simulink model "stand_IM"  (R2024a)
settings: Solver=ode45  StartTime=0.0  StopTime=10.0  RelTol=1e-3  EnableMultiTasking=on
values from neighbouring files (symbols this model uses):
  fn = 50    [stand_final.m]
  pp = 2    [stand_final.m]
  Un = 23.4    [stand_final.m]
libraries: General x35, Math x19, MotorControl x3, Control x3, Basic x2, StateControl x2, Filter x1
settings Model: Creator=hgrabner  LastModifiedBy=adminLab
settings SolverCC: AlgebraicLoopSolver=TrustRegion
settings DataIOCC: LimitDataPoints=on  SaveFormat=Array  SignalLoggingSaveFormat=ModelDataLogs  ReturnWorkspaceOutputs=off
settings OptimizationCC: ExpressionDepthLimit=2147483647  InitFltsAndDblsToZero=on  LifeSpan=inf
settings DebuggingCC: UnderspecifiedInitializationDetection=Classic  MergeDetectMultiDrivingBlocksExec=none  SolverPrmCheckMsg=warning  FcnCallInpInsideContextMsg=warning  UnconnectedInputMsg=warning  UnconnectedOutputMsg=warning  UnconnectedLineMsg=warning  StateNameClashWarn=warning  SFUnexpectedBacktrackingDiag=warning  SFNoUnconditionalDefaultTransitionDiag=warning  SFExecutionAtInitializationDiag=none  ArithmeticOperatorsInVariantConditions=warning
settings HardwareCC: ProdBitPerPointer=32  ProdBitPerSizeT=32  ProdBitPerPtrDiffT=32  ProdLargestAtomicFloat=None  ProdIntDivRoundTo=Undefined  ProdEndianess=Unspecified  ProdWordSize=32  ProdHWDeviceType=32-bit Generic
settings ModelReferenceCC: EnableRefExpFcnMdlSchedulingChecks=on  PropagateSignalLabelsOutOfModel=off
settings SFSimCC: SimUseLocalCustomCode=off  CustomCodeUndefinedFunction=UseInterfaceOnly
settings RTWCC: RTWUseLocalCustomCode=off  GPUComputeCapability=3.5  DLArmComputeVersion=19.05
settings CodeAppCC: StateflowObjectComments=on
settings GRTTargetCC: TargetLangStandard=C89/C90 (ANSI)  CombineOutputUpdateFcns=off  GRTInterface=on
settings ConfigComp: CovMetricSettings=dw  CovSaveCumulativeToWorkspaceVar=on  CovSaveSingleToWorkspaceVar=on  CovExternalEMLEnable=off

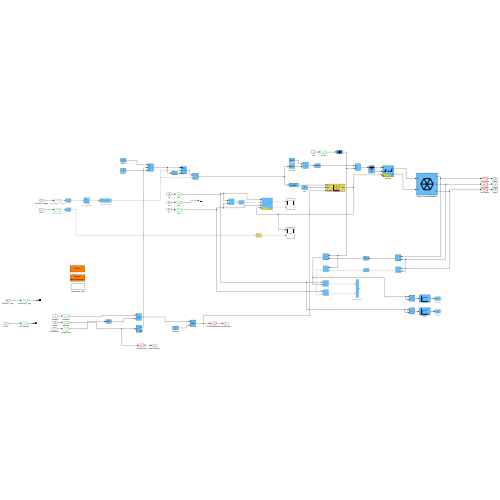
[thumbnail: Simulink's stored preview of the top-level diagram]
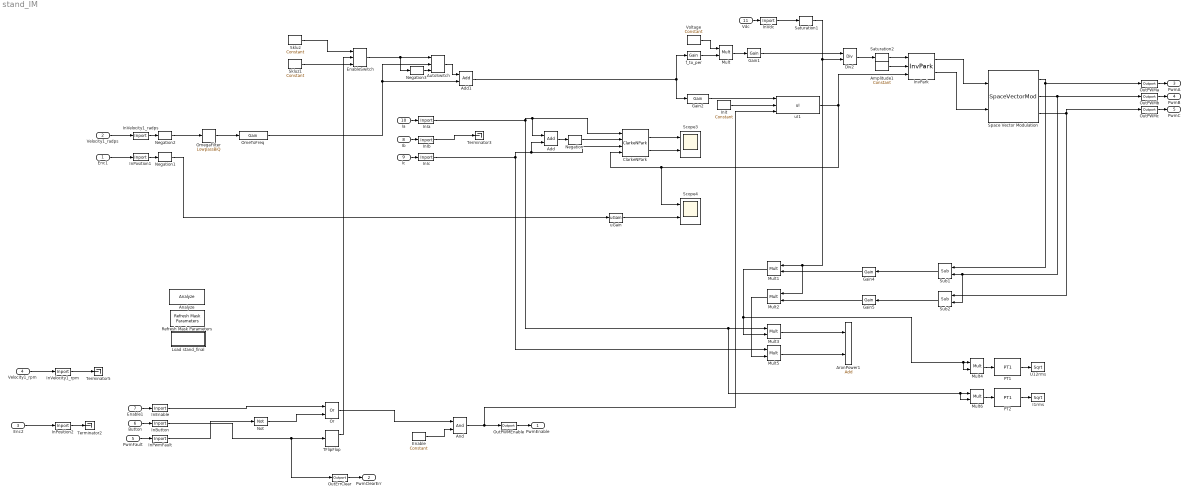
== system stand_IM ==
  Enc1 : Inport
  Velocity1_radps : Inport  Port=2
  Enc2 : Inport  Port=3
  Velocity1_rpm : Inport  Port=4
  PwmFault : Inport  Port=5
  Button : Inport  Port=6
  Enable1 : Inport  Port=7
  Ib : Inport  Port=8
  Ic : Inport  Port=9
  Ia : Inport  Port=10
  Vdc : Inport  Port=11
  Add : Math/Add  M2CAutoParam_UsedImplementation=32 Bit Floating Point  x2c_cfg_enableStaticId=off  x2c_cfg_staticId=1  x2c_cfg_enableCot=off  BlockName=Add
      settings: SourceProductName=X2C Math
  Add1 : Math/Add  M2CAutoParam_UsedImplementation=32 Bit Floating Point  x2c_cfg_enableStaticId=off  x2c_cfg_staticId=1  x2c_cfg_enableCot=off  BlockName=Add
      settings: SourceProductName=X2C Math
  Amplitude1 : General/Constant  Value=0  M2CAutoParam_UsedImplementation=32 Bit Floating Point  x2c_cfg_enableStaticId=off  x2c_cfg_staticId=1  x2c_cfg_enableCot=off  BlockName=Constant
      settings: SourceProductName=X2C General
  Analyze : Basic/Analyze
      settings: SourceProductName=X2C Basic
  And : General/And  M2CAutoParam_UsedImplementation=Boolean  x2c_cfg_enableStaticId=off  x2c_cfg_staticId=1  x2c_cfg_enableCot=off  BlockName=And
      settings: SourceProductName=X2C General
  AronPower1 : Math/Add  M2CAutoParam_UsedImplementation=32 Bit Floating Point  x2c_cfg_enableStaticId=off  x2c_cfg_staticId=1  x2c_cfg_enableCot=off  BlockName=Add
      settings: SourceProductName=X2C Math
  AutoSwitch : General/AutoSwitch  Thresh_up=0.1  Thresh_down=-0.1  M2CAutoParam_UsedImplementation=32 Bit Floating Point  x2c_cfg_enableStaticId=off  x2c_cfg_staticId=1  x2c_cfg_enableCot=off  BlockName=AutoSwitch
      settings: SourceProductName=X2C General
  ClarkeNPark : MotorControl/ClarkeNPark  M2CAutoParam_UsedImplementation=32 Bit Floating Point  x2c_cfg_enableStaticId=off  x2c_cfg_staticId=1  x2c_cfg_enableCot=off  BlockName=ClarkeNPark
      settings: SourceProductName=X2C MotorControl
  Div2 : Math/Div  M2CAutoParam_UsedImplementation=32 Bit Floating Point  x2c_cfg_enableStaticId=off  x2c_cfg_staticId=1  x2c_cfg_enableCot=off  BlockName=Div
      settings: SourceProductName=X2C Math
  Enable : General/Constant  Value=1  M2CAutoParam_UsedImplementation=Boolean  x2c_cfg_enableStaticId=off  x2c_cfg_staticId=1  x2c_cfg_enableCot=off  BlockName=Constant
      settings: SourceProductName=X2C General
  EnableSwitch : StateControl/EnableSwitch  M2CAutoParam_UsedImplementation=32 Bit Floating Point  x2c_cfg_enableStaticId=off  x2c_cfg_staticId=1  x2c_cfg_enableCot=off  BlockName=EnableSwitch
      settings: SourceProductName=X2C StateControl
  Gain1 : General/Gain  Gain=1.4142  M2CAutoParam_UsedImplementation=32 Bit Floating Point  x2c_cfg_enableStaticId=off  x2c_cfg_staticId=1  x2c_cfg_enableCot=off  BlockName=Gain
      settings: SourceProductName=X2C General
  Gain2 : General/Gain  Gain=2*pi  M2CAutoParam_UsedImplementation=32 Bit Floating Point  x2c_cfg_enableStaticId=off  x2c_cfg_staticId=1  x2c_cfg_enableCot=off  BlockName=Gain
      settings: SourceProductName=X2C General
  Gain4 : General/Gain  Gain=0.5  M2CAutoParam_UsedImplementation=32 Bit Floating Point  x2c_cfg_enableStaticId=off  x2c_cfg_staticId=1  x2c_cfg_enableCot=off  BlockName=Gain
      settings: SourceProductName=X2C General
  Gain5 : General/Gain  Gain=0.5  M2CAutoParam_UsedImplementation=32 Bit Floating Point  x2c_cfg_enableStaticId=off  x2c_cfg_staticId=1  x2c_cfg_enableCot=off  BlockName=Gain
      settings: SourceProductName=X2C General
  I1rms : Math/Sqrt  M2CAutoParam_UsedImplementation=32 Bit Floating Point  x2c_cfg_enableStaticId=off  x2c_cfg_staticId=1  x2c_cfg_enableCot=off  BlockName=Sqrt
      settings: SourceProductName=X2C Math
  InButton : General/Inport  DataType=bool  ts_fact=1.0  x2c_cfg_enableStaticId=off  x2c_cfg_staticId=0  BlockName=Inport  gain=1  offset=0
      settings: SourceProductName=X2C General
  InEnable : General/Inport  DataType=bool  ts_fact=1.0  x2c_cfg_enableStaticId=off  x2c_cfg_staticId=0  BlockName=Inport  gain=1  offset=0
      settings: SourceProductName=X2C General
  InIa : General/Inport  DataType=float32  ts_fact=1.0  x2c_cfg_enableStaticId=off  x2c_cfg_staticId=0  BlockName=Inport  gain=1  offset=0
      settings: SourceProductName=X2C General
  InIb : General/Inport  DataType=float32  ts_fact=1.0  x2c_cfg_enableStaticId=off  x2c_cfg_staticId=0  BlockName=Inport  gain=1  offset=0
      settings: SourceProductName=X2C General
  InIc : General/Inport  DataType=float32  ts_fact=1.0  x2c_cfg_enableStaticId=off  x2c_cfg_staticId=0  BlockName=Inport  gain=1  offset=0
      settings: SourceProductName=X2C General
  InPosition1 : General/Inport  DataType=float32  ts_fact=20  x2c_cfg_enableStaticId=off  x2c_cfg_staticId=0  BlockName=Inport  gain=1  offset=0
      settings: SourceProductName=X2C General
  InPosition2 : General/Inport  DataType=float32  ts_fact=1.0  x2c_cfg_enableStaticId=off  x2c_cfg_staticId=0  BlockName=Inport  gain=1  offset=0
      settings: SourceProductName=X2C General
  InPwmFault : General/Inport  DataType=bool  ts_fact=1.0  x2c_cfg_enableStaticId=off  x2c_cfg_staticId=0  BlockName=Inport  gain=1  offset=0
      settings: SourceProductName=X2C General
  InVdc : General/Inport  DataType=float32  ts_fact=1.0  x2c_cfg_enableStaticId=off  x2c_cfg_staticId=0  BlockName=Inport  gain=1  offset=0
      settings: SourceProductName=X2C General
  InVelocity1_radps : General/Inport  DataType=float32  ts_fact=20  x2c_cfg_enableStaticId=off  x2c_cfg_staticId=0  BlockName=Inport  gain=1  offset=0
      settings: SourceProductName=X2C General
  InVelocity1_rpm : General/Inport  DataType=float32  ts_fact=1.0  x2c_cfg_enableStaticId=off  x2c_cfg_staticId=0  BlockName=Inport  gain=1  offset=0
      settings: SourceProductName=X2C General
  Init : General/Constant  Value=0  M2CAutoParam_UsedImplementation=32 Bit Floating Point  x2c_cfg_enableStaticId=off  x2c_cfg_staticId=1  x2c_cfg_enableCot=off  BlockName=Constant
      settings: SourceProductName=X2C General
  InvPark : MotorControl/InvPark  M2CAutoParam_UsedImplementation=32 Bit Floating Point  x2c_cfg_enableStaticId=off  x2c_cfg_staticId=1  x2c_cfg_enableCot=off  BlockName=InvPark
      settings: SourceProductName=X2C MotorControl
  Load stand_final : Subsystem  InitFcn=stand_final
      settings: OpenFcn=stand_final
      mask DialogControl Control2 Prompt: Load stand_final
  Mult{,1..6} (7 alike) : Math/Mult  M2CAutoParam_UsedImplementation=32 Bit Floating Point  x2c_cfg_enableStaticId=off  x2c_cfg_staticId=1  x2c_cfg_enableCot=off  BlockName=Mult
      settings: SourceProductName=X2C Math
  Negation{,1..3} (4 alike) : Math/Negation  M2CAutoParam_UsedImplementation=32 Bit Floating Point  x2c_cfg_enableStaticId=off  x2c_cfg_staticId=1  x2c_cfg_enableCot=off  BlockName=Negation
      settings: SourceProductName=X2C Math
  Not : General/Not  M2CAutoParam_UsedImplementation=Boolean  x2c_cfg_enableStaticId=off  x2c_cfg_staticId=1  x2c_cfg_enableCot=off  BlockName=Not
      settings: SourceProductName=X2C General
  OmeToFreq : General/Gain  Gain=2/2/pi  M2CAutoParam_UsedImplementation=32 Bit Floating Point  x2c_cfg_enableStaticId=off  x2c_cfg_staticId=1  x2c_cfg_enableCot=off  BlockName=Gain
      settings: SourceProductName=X2C General
  OmegaFilter : Filter/LowpassBiQ  characteristic=Chebyshev II  fc=200  rp=1  rs=20  ts_fact=20  M2CAutoParam_UsedImplementation=32 Bit Floating Point  x2c_cfg_enableStaticId=off  x2c_cfg_staticId=1  x2c_cfg_enableCot=off  BlockName=LowpassBiQ
      settings: SourceProductName=X2C Filter
  Or : General/Or  M2CAutoParam_UsedImplementation=Boolean  x2c_cfg_enableStaticId=off  x2c_cfg_staticId=1  x2c_cfg_enableCot=off  BlockName=Or
      settings: SourceProductName=X2C General
  OutErrClear : General/Outport  DataType=bool  ts_fact=1.0  x2c_cfg_enableStaticId=off  x2c_cfg_staticId=0  BlockName=Outport  gain=1  offset=0
      settings: SourceProductName=X2C General
  OutPWMEnable : General/Outport  DataType=bool  ts_fact=1.0  x2c_cfg_enableStaticId=off  x2c_cfg_staticId=0  BlockName=Outport  gain=1  offset=0
      settings: SourceProductName=X2C General
  OutPWMa : General/Outport  DataType=float32  ts_fact=1.0  x2c_cfg_enableStaticId=off  x2c_cfg_staticId=0  BlockName=Outport  gain=1  offset=0
      settings: SourceProductName=X2C General
  OutPWMb : General/Outport  DataType=float32  ts_fact=1.0  x2c_cfg_enableStaticId=off  x2c_cfg_staticId=0  BlockName=Outport  gain=1  offset=0
      settings: SourceProductName=X2C General
  OutPWMc : General/Outport  DataType=float32  ts_fact=1.0  x2c_cfg_enableStaticId=off  x2c_cfg_staticId=0  BlockName=Outport  gain=1  offset=0
      settings: SourceProductName=X2C General
  PT1 : Control/PT1  V=1  fc=5  ts_fact=1.0  method=zoh  M2CAutoParam_UsedImplementation=32 Bit Floating Point  x2c_cfg_enableStaticId=off  x2c_cfg_staticId=1  x2c_cfg_enableCot=off  BlockName=PT1
      settings: SourceProductName=X2C Control
  PT2 : Control/PT1  V=1  fc=5  ts_fact=1.0  method=zoh  M2CAutoParam_UsedImplementation=32 Bit Floating Point  x2c_cfg_enableStaticId=off  x2c_cfg_staticId=1  x2c_cfg_enableCot=off  BlockName=PT1
      settings: SourceProductName=X2C Control
  Refresh Mask Parameters : Basic/Refresh Mask Parameters
      settings: SourceProductName=X2C Basic
  Saturation1 : General/Saturation  max=60  min=10  M2CAutoParam_UsedImplementation=32 Bit Floating Point  x2c_cfg_enableStaticId=off  x2c_cfg_staticId=1  x2c_cfg_enableCot=off  BlockName=Saturation
      settings: SourceProductName=X2C General
  Saturation2 : General/Saturation  max=0.999  min=-0.999  M2CAutoParam_UsedImplementation=32 Bit Floating Point  x2c_cfg_enableStaticId=off  x2c_cfg_staticId=1  x2c_cfg_enableCot=off  BlockName=Saturation
      settings: SourceProductName=X2C General
  Scope3 : Scope  NumInputPorts=2
  Scope4 : Scope  NumInputPorts=2
  Skluz : General/Constant  Value=5  M2CAutoParam_UsedImplementation=32 Bit Floating Point  x2c_cfg_enableStaticId=off  x2c_cfg_staticId=1  x2c_cfg_enableCot=off  BlockName=Constant
      settings: SourceProductName=X2C General
  Skluz1 : General/Constant  Value=-4  M2CAutoParam_UsedImplementation=32 Bit Floating Point  x2c_cfg_enableStaticId=off  x2c_cfg_staticId=1  x2c_cfg_enableCot=off  BlockName=Constant
      settings: SourceProductName=X2C General
  Space Vector Modulation : MotorControl/SpaceVectorMod  method=Alternating reversing  M2CAutoParam_UsedImplementation=32 Bit Floating Point  x2c_cfg_enableStaticId=off  x2c_cfg_staticId=1  x2c_cfg_enableCot=off  BlockName=SpaceVectorMod
      settings: SourceProductName=X2C MotorControl
  Sub1 : Math/Sub  M2CAutoParam_UsedImplementation=32 Bit Floating Point  x2c_cfg_enableStaticId=off  x2c_cfg_staticId=1  x2c_cfg_enableCot=off  BlockName=Sub
      settings: SourceProductName=X2C Math
  Sub2 : Math/Sub  M2CAutoParam_UsedImplementation=32 Bit Floating Point  x2c_cfg_enableStaticId=off  x2c_cfg_staticId=1  x2c_cfg_enableCot=off  BlockName=Sub
      settings: SourceProductName=X2C Math
  TFlipFlop : StateControl/TFlipFlop  M2CAutoParam_UsedImplementation=Boolean  x2c_cfg_enableStaticId=off  x2c_cfg_staticId=1  x2c_cfg_enableCot=off  BlockName=TFlipFlop
      settings: SourceProductName=X2C StateControl
  Terminator2 : Terminator
  Terminator3 : Terminator
  Terminator5 : Terminator
  U12rms : Math/Sqrt  M2CAutoParam_UsedImplementation=32 Bit Floating Point  x2c_cfg_enableStaticId=off  x2c_cfg_staticId=1  x2c_cfg_enableCot=off  BlockName=Sqrt
      settings: SourceProductName=X2C Math
  Voltage : General/Constant  Value=Un  M2CAutoParam_UsedImplementation=32 Bit Floating Point  x2c_cfg_enableStaticId=off  x2c_cfg_staticId=1  x2c_cfg_enableCot=off  BlockName=Constant
      settings: SourceProductName=X2C General
  f_to_per : General/Gain  Gain=1/fn  M2CAutoParam_UsedImplementation=32 Bit Floating Point  x2c_cfg_enableStaticId=off  x2c_cfg_staticId=1  x2c_cfg_enableCot=off  BlockName=Gain
      settings: SourceProductName=X2C General
  uGain : General/uGain  Gain=pp  M2CAutoParam_UsedImplementation=32 Bit Floating Point  x2c_cfg_enableStaticId=off  x2c_cfg_staticId=1  x2c_cfg_enableCot=off  BlockName=uGain
      settings: SourceProductName=X2C General
  uI1 : Control/uI  Ki=1  ts_fact=1.0  M2CAutoParam_UsedImplementation=32 Bit Floating Point  x2c_cfg_enableStaticId=off  x2c_cfg_staticId=1  x2c_cfg_enableCot=off  BlockName=uI
      settings: SourceProductName=X2C Control
  PwmEnable : Outport
  PwmClearErr : Outport  Port=2
  PwmA : Outport  Port=3
  PwmB : Outport  Port=4
  PwmC : Outport  Port=5
  wires:
  InIb/1 -> Terminator3/1
  uI1/1 -> InvPark/3, Scope4/1, ClarkeNPark/4
  InvPark/1 -> Space Vector Modulation/1
  Gain1/1 -> Div2/1
  uGain/1 -> Scope4/2
  Gain2/1 -> uI1/1
  InvPark/2 -> Space Vector Modulation/2
  Saturation2/1 -> InvPark/1
  Mult/1 -> Gain1/1
  Voltage/1 -> Mult/1
  Div2/1 -> Saturation2/1
  Init/1 -> uI1/2
  f_to_per/1 -> Mult/2
  ClarkeNPark/1 -> Scope3/1
  ClarkeNPark/2 -> Scope3/2
  Amplitude1/1 -> InvPark/2
  InVdc/1 -> Saturation1/1
  Add/1 -> Negation/1
  Negation/1 -> ClarkeNPark/2
  Space Vector Modulation/2 -> OutPWMb/1, Sub2/2, Sub1/2
  Gain5/1 -> Mult2/2
  Gain4/1 -> Mult1/2
  Mult1/1 -> Mult4/2, Mult4/1, Mult3/2
  Mult2/1 -> Mult5/2
  Saturation1/1 -> Mult1/1, Mult2/1, Div2/2
  Sub2/1 -> Gain5/1
  InIa/1 -> Add/1, ClarkeNPark/1, Mult6/2, Mult6/1, Mult3/1
  Sub1/1 -> Gain4/1
  Space Vector Modulation/1 -> OutPWMa/1, Sub1/1
  Mult5/1 -> AronPower1/2
  Space Vector Modulation/3 -> OutPWMc/1, Sub2/1
  Mult3/1 -> AronPower1/1
  InIc/1 -> Add/2, ClarkeNPark/3, Mult5/1
  Negation1/1 -> uGain/1
  Mult4/1 -> PT1/1
  PT1/1 -> U12rms/1
  PT2/1 -> I1rms/1
  Mult6/1 -> PT2/1
  InButton/1 -> OutErrClear/1, TFlipFlop/1
  InPwmFault/1 -> Not/1
  Not/1 -> Or/2
  InEnable/1 -> Or/1
  Or/1 -> And/1
  And/1 -> OutPWMEnable/1, uI1/3
  OmeToFreq/1 -> AutoSwitch/2, Add1/2
  EnableSwitch/1 -> AutoSwitch/1, Negation3/1
  AutoSwitch/1 -> Add1/1
  Negation3/1 -> AutoSwitch/3
  Add1/1 -> Gain2/1, f_to_per/1
  Enable/1 -> And/2
  TFlipFlop/1 -> EnableSwitch/2
  Skluz/1 -> EnableSwitch/1
  Skluz1/1 -> EnableSwitch/3
  Velocity1_radps/1 -> InVelocity1_radps/1
  InPosition1/1 -> Negation1/1
  Enc1/1 -> InPosition1/1
  InVelocity1_rpm/1 -> Terminator5/1
  Enc2/1 -> InPosition2/1
  Velocity1_rpm/1 -> InVelocity1_rpm/1
  InPosition2/1 -> Terminator2/1
  PwmFault/1 -> InPwmFault/1
  Enable1/1 -> InEnable/1
  Button/1 -> InButton/1
  Ic/1 -> InIc/1
  Ib/1 -> InIb/1
  Ia/1 -> InIa/1
  Vdc/1 -> InVdc/1
  OutErrClear/1 -> PwmClearErr/1
  OutPWMEnable/1 -> PwmEnable/1
  OutPWMb/1 -> PwmB/1
  OutPWMc/1 -> PwmC/1
  OutPWMa/1 -> PwmA/1
  InVelocity1_radps/1 -> Negation2/1
  Negation2/1 -> OmegaFilter/1
  OmegaFilter/1 -> OmeToFreq/1

== system stand_IM/Load stand_final ==
